simulink model "skyhookidealMRcom"  (R2016a)
settings: Solver=VariableStepAuto  StartTime=0.0  StopTime=10.0  RelTol=1e-3
undefined symbols (not defined in the file): b1, k1, k2, m1, m2
settings Model: Creator=mm395  LastModifiedBy=mm395

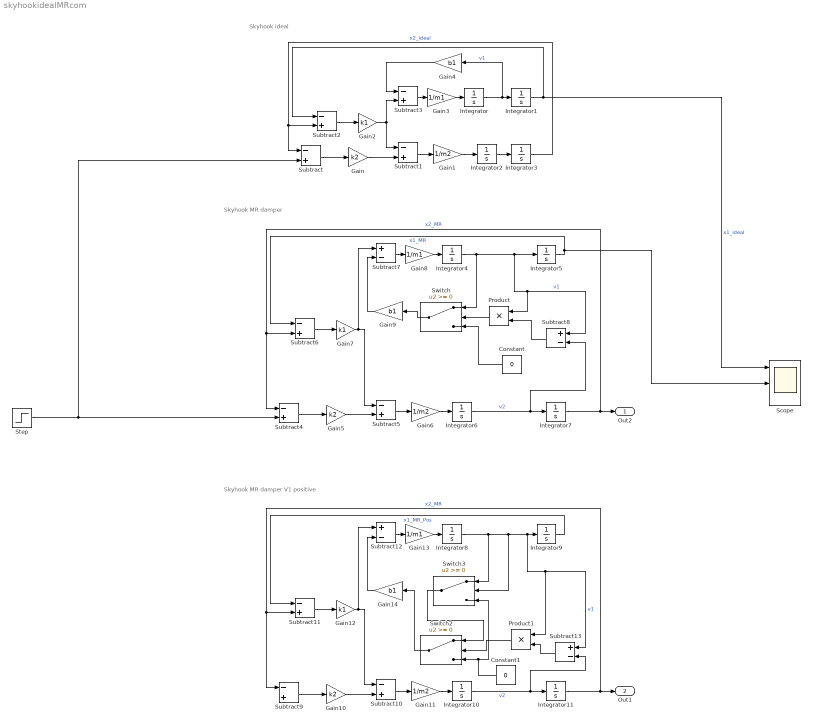
== system skyhookidealMRcom ==
  note: Skyhook ideal
  note: Skyhook MR damper
  note: Skyhook MR damper V1 positive
  Constant : Constant  Value=0
  Constant1 : Constant  Value=0
  Gain : Gain  Gain=k2
  Gain1 : Gain  Gain=1/m2
  Gain10 : Gain  Gain=k2
  Gain11 : Gain  Gain=1/m2
  Gain12 : Gain  Gain=k1
  Gain13 : Gain  Gain=1/m1
  Gain14 : Gain  Gain=b1
  Gain2 : Gain  Gain=k1
  Gain3 : Gain  Gain=1/m1
  Gain4 : Gain  Gain=b1
  Gain5 : Gain  Gain=k2
  Gain6 : Gain  Gain=1/m2
  Gain7 : Gain  Gain=k1
  Gain8 : Gain  Gain=1/m1
  Gain9 : Gain  Gain=b1
  Integrator{,1..11} (12 alike) : Integrator
  Product : Product
  Product1 : Product
  Scope : Scope  NumInputPorts=3
  Step : Step  SampleTime=0  ZeroCross=off
  Subtract{,1..6,9..11} (10 alike) : Sum  Inputs=-+
  Subtract{7..8,12..13} (4 alike) : Sum  Inputs=+-
  Switch : Switch  ZeroCross=off
  Switch2 : Switch  ZeroCross=off
  Switch3 : Switch  ZeroCross=off
  Out2 : Outport
  Out1 : Outport  Port=2
  wires:
  Subtract/1 -> Gain/1
  Gain/1 -> Subtract1/2
  Subtract1/1 -> Gain1/1
  Integrator3/1 -> Subtract/1, Subtract2/2  "x2_ideal"
  Subtract2/1 -> Gain2/1
  Gain2/1 -> Subtract1/1, Subtract3/2
  Subtract3/1 -> Gain3/1
  Gain3/1 -> Integrator/1
  Integrator/1 -> Gain4/1, Integrator1/1  "v1"
  Integrator2/1 -> Integrator3/1
  Gain1/1 -> Integrator2/1
  Integrator1/1 -> Subtract2/1, Scope/1  "x1_ideal"
  Gain4/1 -> Subtract3/1
  Subtract4/1 -> Gain5/1
  Gain5/1 -> Subtract5/2
  Subtract5/1 -> Gain6/1
  Integrator7/1 -> Out2/1, Subtract4/1, Subtract6/2  "x2_MR"
  Subtract6/1 -> Gain7/1
  Gain7/1 -> Subtract7/1, Subtract5/1
  Subtract7/1 -> Gain8/1
  Gain8/1 -> Integrator4/1
  Integrator4/1 -> Switch/1, Integrator5/1, Subtract8/1, Product/1  "v1"
  Integrator6/1 -> Subtract8/2, Integrator7/1  "v2"
  Gain6/1 -> Integrator6/1
  Integrator5/1 -> Scope/2, Subtract6/1  "x1_MR"
  Subtract8/1 -> Product/2
  Product/1 -> Switch/2
  Switch/1 -> Gain9/1
  Gain9/1 -> Subtract7/2
  Constant/1 -> Switch/3
  Step/1 -> Subtract/2, Subtract4/2
  Subtract9/1 -> Gain10/1
  Gain10/1 -> Subtract10/2
  Subtract10/1 -> Gain11/1
  Integrator11/1 -> Out1/1, Subtract9/1, Subtract11/2  "x2_MR"
  Subtract11/1 -> Gain12/1
  Gain12/1 -> Subtract12/1, Subtract10/1
  Subtract12/1 -> Gain13/1
  Gain13/1 -> Integrator8/1
  Integrator8/1 -> Switch3/1, Switch3/2, Product1/1, Subtract13/1, Integrator9/1  "v1"
  Integrator10/1 -> Subtract13/2, Integrator11/1  "v2"
  Gain11/1 -> Integrator10/1
  Integrator9/1 -> Subtract11/1  "x1_MR_Pos"
  Subtract13/1 -> Product1/2
  Product1/1 -> Switch2/2
  Switch2/1 -> Gain14/1
  Gain14/1 -> Subtract12/2
  Constant1/1 -> Switch3/3, Switch2/3
  Switch3/1 -> Switch2/1
